simulink model "NewSpacecraft"  (R2020b)
settings: Solver=VariableStepAuto  StartTime=0.0  StopTime=10.0  RelTol=1e-3
undefined symbols (not defined in the file or in its folder): sim_constants
libraries: vrlib x2
settings Model: Creator=newpo  LastModifiedBy=newpo

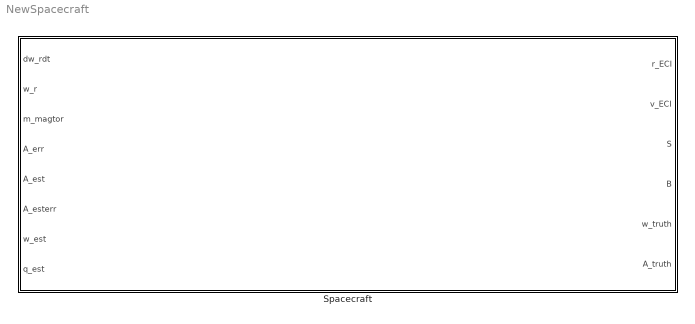
== system NewSpacecraft ==
  Spacecraft : Subsystem

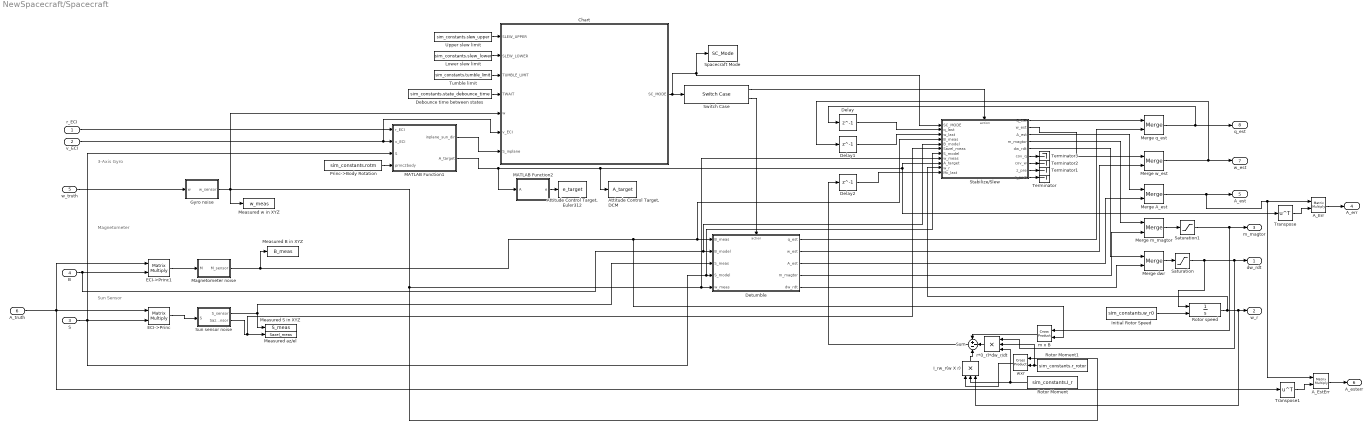
== system NewSpacecraft/Spacecraft ==
  note: Sun Sensor
  note: Magnetometer
  note: 3-Axis Gyro
  r_ECI : Inport
  v_ECI : Inport  Port=2
  S : Inport  Port=3
  B : Inport  Port=4
  w_truth : Inport  Port=5
  A_truth : Inport  Port=6
  A_Err : Product  Multiplication=Matrix(*)
  A_EstErr : Product  Multiplication=Matrix(*)
  "Attitude Control Target, DCM" : ToWorkspace  VariableName=A_target  SaveFormat=Timeseries  SampleTime=-1
  "Attitude Control Target, Euler312" : ToWorkspace  VariableName=e_target  SaveFormat=Timeseries  SampleTime=-1
  Chart : Stateflow chart  TreatAsAtomicUnit=on
  Debounce time between states : Constant  Value=sim_constants.state_debounce_time
  Delay : Delay  DelayLength=1  InitialCondition=sim_constants.q0
  Delay1 : Delay  DelayLength=1  InitialCondition=sim_constants.angvel0
  Delay2 : Delay  DelayLength=1  InitialCondition=[0;0;0]
  Detumble : Subsystem  TreatAsAtomicUnit=on
  ECI->Princ : Product  Multiplication=Matrix(*)
  ECI->Princ1 : Product  Multiplication=Matrix(*)
  Gyro noise : Subsystem
  I_rw_r(w X r) : Product  Inputs=3
  Initial Rotor Speed : Constant  Value=sim_constants.w_r0
  Lower slew limit : Constant  Value=sim_constants.slew_lower
  MATLAB Function1 : MATLAB Function  TreatAsAtomicUnit=on
  MATLAB Function2 : MATLAB Function  TreatAsAtomicUnit=on
  Magnetometer noise : Subsystem
  Measured B in XYZ : ToWorkspace  VariableName=B_meas  SaveFormat=Timeseries  SampleTime=-1
  Measured S in XYZ : ToWorkspace  VariableName=S_meas  SaveFormat=Timeseries  SampleTime=-1
  Measured az/el : ToWorkspace  VariableName=Sazel_meas  SaveFormat=Timeseries  SampleTime=-1
  Measured w in XYZ : ToWorkspace  VariableName=w_meas  SaveFormat=Timeseries  SampleTime=-1
  Merge A_est : Merge
  Merge dwr : Merge
  Merge m_magtor : Merge
  Merge q_est : Merge
  Merge w_est : Merge
  Princ->Body Rotation : Constant  Value=sim_constants.rotm
  Rotor Moment : Constant  Value=sim_constants.I_r
  Rotor Moment1 : Constant  Value=sim_constants.r_rotor
  Rotor speed : Integrator  InitialConditionSource=external  LimitOutput=on  UpperSaturationLimit=sim_constants.w_rmax  LowerSaturationLimit=-sim_constants.w_rmax
  Saturation : Saturate  UpperLimit=sim_constants.dw_rdtmax  LowerLimit=-sim_constants.dw_rdtmax
  Saturation1 : Saturate  UpperLimit=sim_constants.m_magtor_max  LowerLimit=-sim_constants.m_magtor_max
  Spacecraft Mode : ToWorkspace  VariableName=SC_Mode  SaveFormat=Timeseries  SampleTime=-1
  Stabilize/Slew : Subsystem  TreatAsAtomicUnit=on
  Sum : Sum  Inputs=+--
  Sun sensor noise : Subsystem
  Switch Case : SwitchCase  CaseConditions={[SCModeEnum.STABILIZE,SCModeEnum.SLEW],SCModeEnum.DETUMBLE}  ShowDefaultCase=off
  Terminator{,1..3} (4 alike) : Terminator
  Transpose : Math  Operator=transpose  SaturateOnIntegerOverflow=on
  Transpose1 : Math  Operator=transpose  SaturateOnIntegerOverflow=on
  Tumble limit : Constant  Value=sim_constants.tumble_limit
  Upper slew limit : Constant  Value=sim_constants.slew_upper
  m x B : vrlib/Utilities/Cross Product
  r*(I_r)*dw_r/dt : Product  Inputs=3
  wxr : vrlib/Utilities/Cross Product
  dw_rdt : Outport
  w_r : Outport  Port=2
  m_magtor : Outport  Port=3
  A_err : Outport  Port=4
  A_est : Outport  Port=5
  A_esterr : Outport  Port=6
  w_est : Outport  Port=7
  q_est : Outport  Port=8
  wires:
  Gyro noise/1(w_sensor) -> Chart/5(w), wxr/1, Stabilize/Slew/8(w_meas), Detumble/5(w_meas), Measured w in XYZ/1
  B/1 -> Stabilize/Slew/5(B_model), Detumble/2(B_model), ECI->Princ1/2
  Sun sensor noise/1(S_sensor) -> Measured S in XYZ/1, Detumble/3(S_meas)
  w_truth/1 -> Gyro noise/1(w)
  Sun sensor noise/2(Sazel_sensor) -> Stabilize/Slew/6(Sazel_meas), Measured az/el/1
  A_truth/1 -> Transpose1/1, ECI->Princ1/1, ECI->Princ/1
  ECI->Princ/1 -> Sun sensor noise/1(S)
  ECI->Princ1/1 -> Magnetometer noise/1(M)
  Princ->Body Rotation/1 -> MATLAB Function1/4(princ2body)
  MATLAB Function1/1(inplane_sun_dir) -> Chart/7(S_inplane)
  v_ECI/1 -> Chart/6(v_ECI), MATLAB Function1/2(v_ECI)
  r_ECI/1 -> MATLAB Function1/1(r_ECI)
  Chart/1(SC_MODE) -> Spacecraft Mode/1, Stabilize/Slew/1(SC_MODE), Switch Case/1
  Switch Case/2 -> Detumble/Action
  Magnetometer noise/1(M_sensor) -> m x B/2, Stabilize/Slew/4(B_meas), Detumble/1(B_meas), Measured B in XYZ/1
  S/1 -> Stabilize/Slew/7(S_model), Detumble/4(S_model), MATLAB Function1/3(S), ECI->Princ/2
  Switch Case/1 -> Stabilize/Slew/Action
  Merge q_est/1 -> Delay/1, q_est/1
  Delay/1 -> Stabilize/Slew/2(q_last)
  Detumble/1(q_est) -> Merge q_est/2
  Stabilize/Slew/1(q_est) -> Merge q_est/1
  Merge w_est/1 -> Delay1/1, w_est/1
  Delay1/1 -> Stabilize/Slew/3(w_last)
  Detumble/2(w_est) -> Merge w_est/2
  Stabilize/Slew/2(w_est) -> Merge w_est/1
  Rotor speed/1 -> I_rw_r(w X r)/3, w_r/1, Stabilize/Slew/10(w_r)
  Initial Rotor Speed/1 -> Rotor speed/2
  Merge dwr/1 -> Saturation/1
  Merge A_est/1 -> A_EstErr/1, A_Err/1, A_est/1
  Stabilize/Slew/3(A_est) -> Merge A_est/1
  Stabilize/Slew/4(m_magtor) -> Merge m_magtor/1
  Stabilize/Slew/5(dw_rdt) -> Merge dwr/1
  Detumble/3(A_est) -> Merge A_est/2
  Detumble/4(m_magtor) -> Merge m_magtor/2
  Detumble/5(dw_rdt) -> Merge dwr/2
  MATLAB Function1/2(A_target) -> MATLAB Function2/1(A), "Attitude Control Target, DCM"/1, Transpose/1, Stabilize/Slew/9(A_target)
  Stabilize/Slew/9(z_post) -> Terminator/1
  Stabilize/Slew/8(z_pre) -> Terminator1/1
  Stabilize/Slew/7(cov_w) -> Terminator2/1
  Stabilize/Slew/6(cov_q) -> Terminator3/1
  Transpose/1 -> A_Err/2
  A_Err/1 -> A_err/1
  Transpose1/1 -> A_EstErr/2
  A_EstErr/1 -> A_esterr/1
  Upper slew limit/1 -> Chart/1(SLEW_UPPER)
  Lower slew limit/1 -> Chart/2(SLEW_LOWER)
  Tumble limit/1 -> Chart/3(TUMBLE_LIMIT)
  Debounce time between states/1 -> Chart/4(TWAIT)
  MATLAB Function2/1(e) -> "Attitude Control Target, Euler312"/1
  Saturation/1 -> Rotor speed/1, r*(I_r)*dw_r/dt/1, dw_rdt/1
  Merge m_magtor/1 -> Saturation1/1
  Saturation1/1 -> m x B/1, m_magtor/1
  m x B/1 -> Sum/1
  Rotor Moment1/1 -> r*(I_r)*dw_r/dt/2, wxr/2
  Rotor Moment/1 -> I_rw_r(w X r)/2, r*(I_r)*dw_r/dt/3
  I_rw_r(w X r)/1 -> Sum/3
  wxr/1 -> I_rw_r(w X r)/1
  r*(I_r)*dw_r/dt/1 -> Sum/2
  Sum/1 -> Delay2/1
  Delay2/1 -> Stabilize/Slew/11(Mc_last)

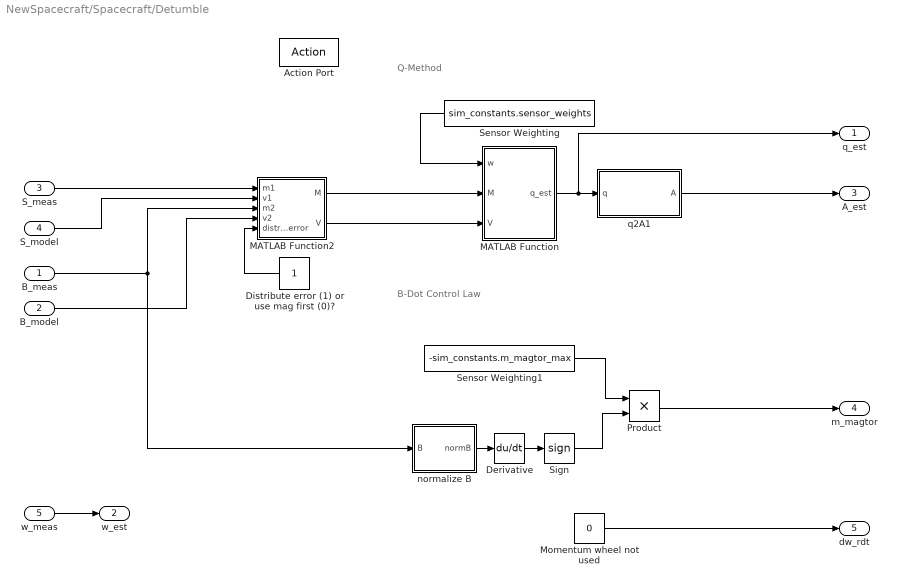
== system NewSpacecraft/Spacecraft/Detumble ==
  note: B-Dot Control Law
  note: Q-Method
  B_meas : Inport
  B_model : Inport  Port=2
  S_meas : Inport  Port=3
  S_model : Inport  Port=4
  w_meas : Inport  Port=5
  Action Port : ActionPort
  Derivative : Derivative  CoefficientInTFapproximation=0.1*2*pi*sim_constants.time_step
  Distribute error (1) or use mag first (0)? : Constant
  MATLAB Function : MATLAB Function  TreatAsAtomicUnit=on
  MATLAB Function2 : MATLAB Function  TreatAsAtomicUnit=on
  Momentum wheel not used : Constant  Value=0
  Product : Product
  Sensor Weighting : Constant  Value=sim_constants.sensor_weights
  Sensor Weighting1 : Constant  Value=-sim_constants.m_magtor_max
  Sign : Signum
  normalize B : MATLAB Function  TreatAsAtomicUnit=on
  q2A1 : MATLAB Function  TreatAsAtomicUnit=on
  q_est : Outport
  w_est : Outport  Port=2
  A_est : Outport  Port=3
  m_magtor : Outport  Port=4
  dw_rdt : Outport  Port=5
  wires:
  Sensor Weighting/1 -> MATLAB Function/1(w)
  S_meas/1 -> MATLAB Function2/1(m1)
  MATLAB Function2/2(V) -> MATLAB Function/3(V)
  q2A1/1(A) -> A_est/1
  MATLAB Function/1(q_est) -> q_est/1, q2A1/1(q)
  Distribute error (1) or use mag first (0)?/1 -> MATLAB Function2/5(distribute_error)
  B_meas/1 -> MATLAB Function2/3(m2), normalize B/1(B)
  MATLAB Function2/1(M) -> MATLAB Function/2(M)
  S_model/1 -> MATLAB Function2/2(v1)
  B_model/1 -> MATLAB Function2/4(v2)
  Derivative/1 -> Sign/1
  Sensor Weighting1/1 -> Product/1
  Sign/1 -> Product/2
  Product/1 -> m_magtor/1
  Momentum wheel not used/1 -> dw_rdt/1
  w_meas/1 -> w_est/1
  normalize B/1(normB) -> Derivative/1

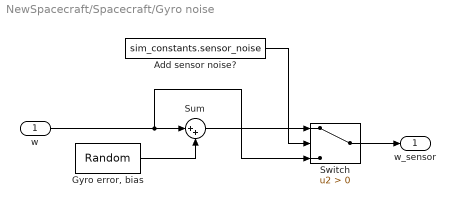
== system NewSpacecraft/Spacecraft/Gyro noise ==
  w : Inport
  Add sensor noise? : Constant  Value=sim_constants.sensor_noise
  "Gyro error, bias" : RandomNumber  Mean=sim_constants.gyro_bias  Variance=sim_constants.gyro_error  Seed=[0, 1, 2]  SampleTime=sim_constants.time_step
  Sum : Sum  Inputs=|++
  Switch : Switch  Criteria=u2 > Threshold
  w_sensor : Outport
  wires:
  "Gyro error, bias"/1 -> Sum/2
  w/1 -> Sum/1, Switch/3
  Switch/1 -> w_sensor/1
  Add sensor noise?/1 -> Switch/2
  Sum/1 -> Switch/1

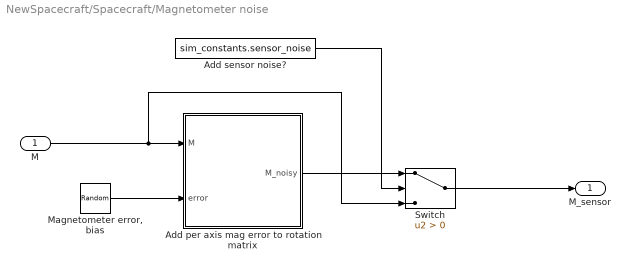
== system NewSpacecraft/Spacecraft/Magnetometer noise ==
  M : Inport
  Add per axis mag error to rotation matrix : MATLAB Function  TreatAsAtomicUnit=on
  Add sensor noise? : Constant  Value=sim_constants.sensor_noise
  "Magnetometer error, bias" : RandomNumber  Mean=sim_constants.mag_bias  Variance=sim_constants.mag_error  Seed=[6, 7, 8]  SampleTime=sim_constants.time_step
  Switch : Switch  Criteria=u2 > Threshold
  M_sensor : Outport
  wires:
  Add per axis mag error to rotation matrix/1(M_noisy) -> Switch/1
  Add sensor noise?/1 -> Switch/2
  M/1 -> Switch/3, Add per axis mag error to rotation matrix/1(M)
  "Magnetometer error, bias"/1 -> Add per axis mag error to rotation matrix/2(error)
  Switch/1 -> M_sensor/1

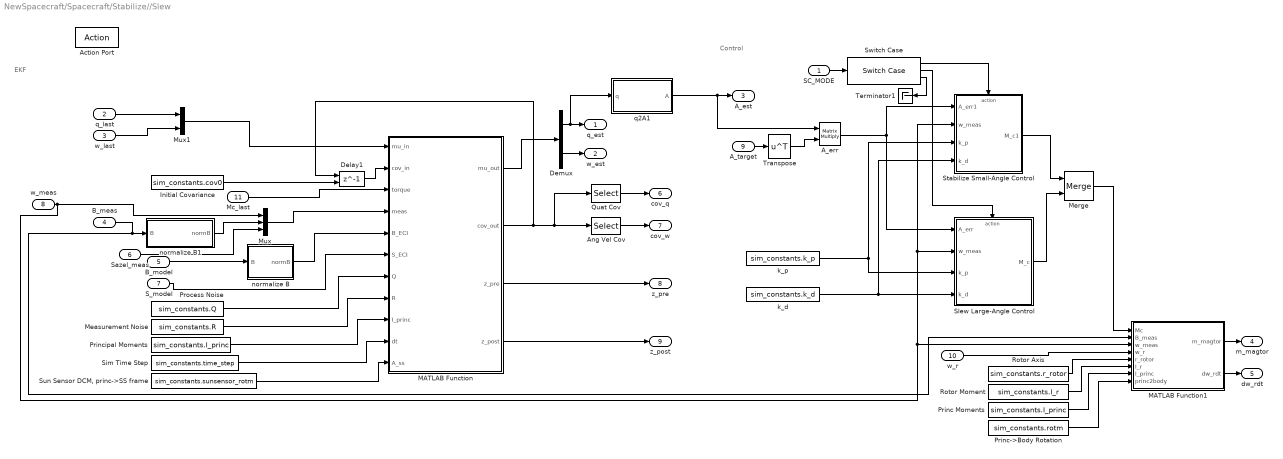
== system NewSpacecraft/Spacecraft/Stabilize//Slew ==
  note: Control
  note: EKF
  SC_MODE : Inport
  q_last : Inport  Port=2
  w_last : Inport  Port=3
  B_meas : Inport  Port=4
  B_model : Inport  Port=5
  Sazel_meas : Inport  Port=6
  S_model : Inport  Port=7
  w_meas : Inport  Port=8
  A_target : Inport  Port=9
  w_r : Inport  Port=10
  Mc_last : Inport  Port=11
  Action Port : ActionPort  InitializeStates=reset
  A_err : Product  Multiplication=Matrix(*)
  Ang Vel Cov : Selector  NumberOfDimensions=2  InputPortWidth=3  IndexOptions=Index vector (dialog),Index vector (dialog)  Indices=5:7,5:7  OutputSizes=1,1
  Delay1 : Delay  DelayLength=1  InitialConditionSource=Input port  InitialCondition=0
      settings: InputPortMap=u0,p4
  Demux : Demux  Outputs=[4, 3]
  Initial Covariance : Constant  Value=sim_constants.cov0
  MATLAB Function : MATLAB Function  TreatAsAtomicUnit=on
  MATLAB Function1 : MATLAB Function  TreatAsAtomicUnit=on
  Measurement Noise : Constant  Value=sim_constants.R
  Merge : Merge
  Mux : Mux  Inputs=3
  Mux1 : Mux  Inputs=2
  Princ Moments : Constant  Value=sim_constants.I_princ
  Princ->Body Rotation : Constant  Value=sim_constants.rotm
  Principal Moments : Constant  Value=sim_constants.I_princ
  Process Noise : Constant  Value=sim_constants.Q
  Quat Cov : Selector  NumberOfDimensions=2  InputPortWidth=3  IndexOptions=Index vector (dialog),Index vector (dialog)  Indices=1:4,1:4  OutputSizes=1,1
  Rotor Axis : Constant  Value=sim_constants.r_rotor
  Rotor Moment : Constant  Value=sim_constants.I_r
  Sim Time Step : Constant  Value=sim_constants.time_step
  Slew Large-Angle Control : Subsystem  TreatAsAtomicUnit=on
  Stabilize Small-Angle Control : Subsystem  TreatAsAtomicUnit=on
  "Sun Sensor DCM, princ->SS frame" : Constant  Value=sim_constants.sunsensor_rotm
  Switch Case : SwitchCase  CaseConditions={SCModeEnum.STABILIZE, SCModeEnum.SLEW}
  Terminator1 : Terminator
  Transpose : Math  Operator=transpose  SaturateOnIntegerOverflow=on
  k_d : Constant  Value=sim_constants.k_d
  k_p : Constant  Value=sim_constants.k_p
  normalize B : MATLAB Function  TreatAsAtomicUnit=on
  normalize B1 : MATLAB Function  TreatAsAtomicUnit=on
  q2A1 : MATLAB Function  TreatAsAtomicUnit=on
  q_est : Outport
  w_est : Outport  Port=2
  A_est : Outport  Port=3
  m_magtor : Outport  Port=4
  dw_rdt : Outport  Port=5
  cov_q : Outport  Port=6
  cov_w : Outport  Port=7
  z_pre : Outport  Port=8
  z_post : Outport  Port=9
  wires:
  "Sun Sensor DCM, princ->SS frame"/1 -> MATLAB Function/11(A_ss)
  Demux/2 -> w_est/1
  Sim Time Step/1 -> MATLAB Function/10(dt)
  Initial Covariance/1 -> Delay1/2
  MATLAB Function/4(z_post) -> z_post/1
  Sazel_meas/1 -> Mux/3
  Measurement Noise/1 -> MATLAB Function/8(R)
  MATLAB Function/3(z_pre) -> z_pre/1
  Ang Vel Cov/1 -> cov_w/1
  Principal Moments/1 -> MATLAB Function/9(I_princ)
  Process Noise/1 -> MATLAB Function/7(Q)
  MATLAB Function/1(mu_out) -> Demux/1
  Demux/1 -> q2A1/1(q), q_est/1
  w_meas/1 -> Mux/1, Stabilize Small-Angle Control/2(w_meas), Slew Large-Angle Control/2(w_meas), MATLAB Function1/3(w_meas)
  S_model/1 -> MATLAB Function/6(S_ECI)
  Mux/1 -> MATLAB Function/4(meas)
  Delay1/1 -> MATLAB Function/2(cov_in)
  B_meas/1 -> MATLAB Function1/2(B_meas), normalize B1/1(B)
  Quat Cov/1 -> cov_q/1
  MATLAB Function/2(cov_out) -> Delay1/1, Quat Cov/1, Ang Vel Cov/1
  B_model/1 -> normalize B/1(B)
  q_last/1 -> Mux1/1
  w_last/1 -> Mux1/2
  Mux1/1 -> MATLAB Function/1(mu_in)
  Mc_last/1 -> MATLAB Function/3(torque)
  Merge/1 -> MATLAB Function1/1(Mc)
  q2A1/1(A) -> A_err/1, A_est/1
  A_target/1 -> Transpose/1
  Transpose/1 -> A_err/2
  SC_MODE/1 -> Switch Case/1
  Switch Case/1 -> Stabilize Small-Angle Control/Action
  Stabilize Small-Angle Control/1(M_c1) -> Merge/1
  Slew Large-Angle Control/1(M_c) -> Merge/2
  MATLAB Function1/1(m_magtor) -> m_magtor/1
  MATLAB Function1/2(dw_rdt) -> dw_rdt/1
  Switch Case/2 -> Slew Large-Angle Control/Action
  A_err/1 -> Slew Large-Angle Control/1(A_err), Stabilize Small-Angle Control/1(A_err1)
  k_p/1 -> Slew Large-Angle Control/3(k_p), Stabilize Small-Angle Control/3(k_p)
  k_d/1 -> Stabilize Small-Angle Control/4(k_d), Slew Large-Angle Control/4(k_d)
  Switch Case/3 -> Terminator1/1
  normalize B/1(normB) -> MATLAB Function/5(B_ECI)
  normalize B1/1(normB) -> Mux/2
  w_r/1 -> MATLAB Function1/4(w_r)
  Rotor Axis/1 -> MATLAB Function1/5(r_rotor)
  Rotor Moment/1 -> MATLAB Function1/6(I_r)
  Princ->Body Rotation/1 -> MATLAB Function1/8(princ2body)
  Princ Moments/1 -> MATLAB Function1/7(I_princ)

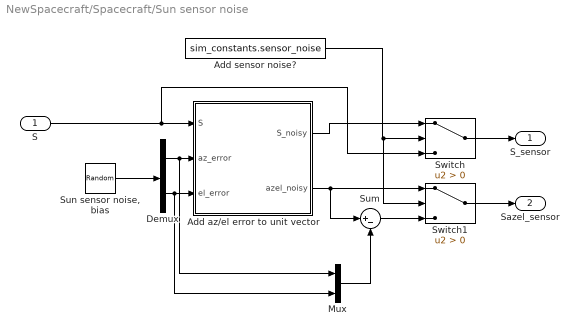
== system NewSpacecraft/Spacecraft/Sun sensor noise ==
  S : Inport
  Add az/el error to unit vector : MATLAB Function  TreatAsAtomicUnit=on
  Add sensor noise? : Constant  Value=sim_constants.sensor_noise
  Demux : Demux  Outputs=2
  Mux : Mux  Inputs=2
  Sum : Sum  Inputs=|+-
  "Sun sensor noise, bias" : RandomNumber  Mean=sim_constants.ss_bias  Variance=sim_constants.ss_error  Seed=[4, 5]  SampleTime=sim_constants.time_step
  Switch : Switch  Criteria=u2 > Threshold
  Switch1 : Switch  Criteria=u2 > Threshold
  S_sensor : Outport
  Sazel_sensor : Outport  Port=2
  wires:
  Demux/1 -> Mux/1, Add az/el error to unit vector/2(az_error)
  Demux/2 -> Mux/2, Add az/el error to unit vector/3(el_error)
  "Sun sensor noise, bias"/1 -> Demux/1
  S/1 -> Switch/3, Add az/el error to unit vector/1(S)
  Switch/1 -> S_sensor/1
  Add az/el error to unit vector/1(S_noisy) -> Switch/1
  Add sensor noise?/1 -> Switch1/2, Switch/2
  Add az/el error to unit vector/2(azel_noisy) -> Sum/1, Switch1/1
  Mux/1 -> Sum/2
  Sum/1 -> Switch1/3
  Switch1/1 -> Sazel_sensor/1

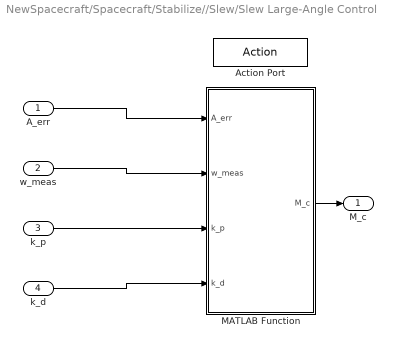
== system NewSpacecraft/Spacecraft/Stabilize//Slew/Slew Large-Angle Control ==
  A_err : Inport
  w_meas : Inport  Port=2
  k_p : Inport  Port=3
  k_d : Inport  Port=4
  Action Port : ActionPort
  MATLAB Function : MATLAB Function  TreatAsAtomicUnit=on
  M_c : Outport
  wires:
  A_err/1 -> MATLAB Function/1(A_err)
  w_meas/1 -> MATLAB Function/2(w_meas)
  k_p/1 -> MATLAB Function/3(k_p)
  k_d/1 -> MATLAB Function/4(k_d)
  MATLAB Function/1(M_c) -> M_c/1

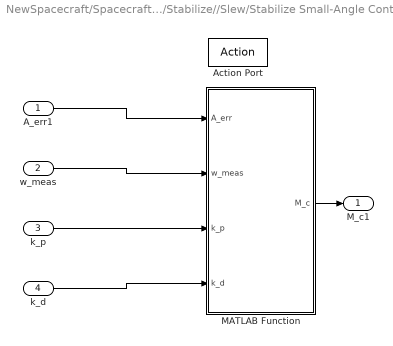
== system NewSpacecraft/Spacecraft/Stabilize//Slew/Stabilize Small-Angle Control ==
  A_err1 : Inport
  w_meas : Inport  Port=2
  k_p : Inport  Port=3
  k_d : Inport  Port=4
  Action Port : ActionPort
  MATLAB Function : MATLAB Function  TreatAsAtomicUnit=on
  M_c1 : Outport
  wires:
  MATLAB Function/1(M_c) -> M_c1/1
  A_err1/1 -> MATLAB Function/1(A_err)
  w_meas/1 -> MATLAB Function/2(w_meas)
  k_d/1 -> MATLAB Function/4(k_d)
  k_p/1 -> MATLAB Function/3(k_p)

== matlab function NewSpacecraft/Spacecraft/MATLAB Function1 ==
  data: inplane_sun_dir output; r_ECI input; A_target output; v_ECI input; S input; princ2body input
function [inplane_sun_dir, A_target] = target_attitude(r_ECI, v_ECI, S, princ2body)
    % Calculate in-plane sun direction
    h = cross(r_ECI, v_ECI); % angular momentum vector, normal to orbital plane
    h = h/norm(h); % unitize
    inplane_sun_dir = S - dot(h,S)*h; % get in-plane sun direction
    if all(abs(inplane_sun_dir) < 1E-6)% if sun direction is perpendicular to orbital plane 
        inplane_sun_dir = r_ECI/norm(r_ECI); % just assume sun is in radial direction
    else
        inplane_sun_dir = inplane_sun_dir/norm(inplane_sun_dir);
    end
    A_body2ECI = zeros(3);
    if dot(v_ECI, S) < 0 % if moving away from the sun
        A_body2ECI(:,1) = h; % align body x axis with orbit plane normal
        A_body2ECI(:,3) = -inplane_sun_dir; % align body z to be along projection of -S in orbit plane (SRP thrusting in-plane)
        A_body2ECI(:,2) = cross( A_body2ECI(:,2) ,  A_body2ECI(:,3) ); % y completes triad
    else
        A_body2ECI(:,1) = h; % align body x axis with orbit plane normal
        A_body2ECI(:,2) = inplane_sun_dir; % align body y to be along projection of S in orbit plane (no thrusting)
        A_body2ECI(:,3) = cross( A_body2ECI(:,1) ,  A_body2ECI(:,2) ); % z completes triad
    end
    A_target = A_body2ECI*(princ2body.'); % princ->body->ECI
    A_target = A_target.'; % ECI->Princ(target)
end

== matlab function NewSpacecraft/Spacecraft/Detumble/MATLAB Function2 ==
  data: m1 input; v1 input; M output; m2 input; v2 input; V output; distribute_error input
function [M, V] = makeMV(m1, v1, m2, v2, distribute_error)

    if distribute_error
        m1_av = (m1 + m2)/2;
        m2_av = (m1 - m2)/2;
        m1 = m1_av; m2 = m2_av;
        
        v1_av = (v1 + v2)/2;
        v2_av = (v1 - v2)/2;
        v1 = v1_av; v2 = v2_av;
    end
        
    q = cross(m1,m2);
    q = q/norm(q);
    r = cross(m1,q);
    M = [m1, q, r];

    qv = cross(v1,v2);
    qv = qv/norm(qv);
    rv = cross(v1,qv);
    V = [v1, qv, rv];

end

== matlab function NewSpacecraft/Spacecraft/Stabilize//Slew/MATLAB Function ==
  data: mu_in input; mu_out output; cov_in input; torque input; meas input; B_ECI input; S_ECI input; Q input; R input; I_princ input; dt input; cov_out output; z_pre output; z_post output; A_ss input
%% satEKF
% Extended Kalman filter for satellite attitude state estimation.
% mu_in : the current estimated state mean, in the form
%           (q, w, bw, bB, bS)^T
%           where q is the quaternion, w is the principal axes angular
%           velocity, bw is the gyroscopic sensor bias, bB is the magnetic
%           sensor bias, and bS is the azimuth/elevation sun sensor bias.
% cov_in : the current covariance matrix
% torque : the input torque to the system at the current time step
% meas : the measurement of the current state
% B_ECI : the modeled magnetic field vector in inertial coordinates at current time
% S_ECI: the modeled sun-pointing vector in intertial coordinates at current time 
% Q : the process noise matrix
% R : the measurement noise matrix
% I_princ : the principal moments of inertia corresponding to principal XYZ
% dt : the time step
% A_ss : the rotation from principal axes to sun sensor frame
function [mu_out, cov_out, z_pre, z_post] = satEKF_nobias(mu_in, cov_in, torque, meas, B_ECI, S_ECI, Q, R, I_princ, dt, A_ss)
    q = mu_in(1:4); % quaternion
    q = q/norm(q);
    w = mu_in(5:7); % angular velocity in princ
    
    At = A(q,w,I_princ,dt);
    %% Predict - use non-linear function to predict mean, linearized info for cov
    mu_p = f(mu_in,torque,I_princ,dt); % get predicted state from non-linear eq
    cov_p = At*cov_in*(At.') + Q;
    A_p = q2A(mu_p(1:4)/norm(mu_p(1:4))); % get rotation matrix of predicted state
    meas_p = g(mu_p,A_p*B_ECI,A_p*S_ECI,A_ss); % predicted measurement
    z_pre = z(meas, meas_p); % pre-fit residual (diff between real and predicted)
    %% Update - use predicted states to compute Kalman gain and final update
    % Update state using sensitivity matrix
    q_p = mu_p(1:4)/norm(mu_p(1:4));
    Ct = C(q_p,q2A(q_p),B_ECI,S_ECI,A_ss); % Sensitivity matrix
    K = cov_p*(Ct.')/(Ct*cov_p*(Ct.') + R) ; % Kalman Gain
    mu_out = mu_p + K*z_pre;
    T = (eye(7) - K*Ct);
    cov_out = T*cov_p*(T.') + K*R*(K.');
    A_f = q2A(mu_out(1:4)/norm(mu_out(1:4)));
    z_post = z(meas, g(mu_out,A_f*B_ECI,A_f*S_ECI,A_ss));  % post-fit residual (diff between real and estimated)
end
% Helper Functions
    function O = Omega(w)
        % Returns Omega(w), the rate relation such that dw/dt = 0.5*Omega*q
        O = [0 w(3) -w(2) w(1);
             -w(3) 0 w(1) w(2);
             w(2) -w(1) 0 w(3);
             -w(1) -w(2) -w(3) 0];
    end
    function L = Lambda(q)
        % Returns Lambda(q), the rate relation such that dw/dt = 0.5*Lambda*w
        L = [q(4) -q(3) q(2);
             q(3) q(4) -q(1);
             -q(2) q(1) q(4);
             -q(1) -q(2) -q(3) ];
    end
    function D = Delta(w,I)
        % Returns Delta(w), the partial derivative of the Euler equations
        % wrt angular velocity.
        D = [0 (I(2)-I(3))/I(1)*w(3) (I(2)-I(3))/I(1)*w(2);
             (I(3)-I(1))/I(2)*w(3) 0 (I(3)-I(1))/I(2)*w(1);
             (I(1)-I(2))/I(3)*w(2) (I(1)-I(2))/I(3)*w(1) 0 ];
    end
    function G = Gamma(q,V)
        % Returns Gamma(q,V), the partial derivative of A(q)*V wrt to the
        % quaternion, for some vector V in ECI.
        q = q/norm(q);
        qvec = q(1:3);
        a = [-q(2);q(1);-q(4)];
        b = [-q(3);q(4);q(1)];
        c = [q(4); q(3); -q(2)];
        G = 2*[dot(qvec,V) dot(a,V) dot(b,V) dot(c,V);
               dot(-a,V) dot(qvec,V) dot(-c,V) dot(b,V);
               dot(-b,V) dot(c,V) dot(qvec,V) dot(-a,V) ];
    end
    function Mt = M(S)
        Mt = [atan2(S(2),S(1)); acos(S(3))];
    end
    function Mt = Mtilde(S)
        S12 = S(1)^2 + S(2)^2;
        Mt = [-S(2)/S12 S(1)/S12 0; 0 0 -1/sqrt(1-S(3)^2)];
    end
    function xout = f(x,torque,I,dt)
        % Dynamics function such that x_{t+1} = f(x_t, u_t)
        q = x(1:4);
        w = x(5:7);
        s = eye(7); 
        normq = norm(q);
        s(1:4,1:4) = eye(4)/normq;
        xout = s*(x + dt*[0.5*Omega(w)*q ; (torque - cross(w,I.*w))./I]);
    end
    function At = A(q,w,I,dt)
        % Jacobian of dynamics
        normq = norm(q);
        q = q/normq;
        s = eye(7); 
        b = diag((normq^2)*ones(4,1)-(q.^2)); % b = d/dq of (q/norm(q))
        b(1,2:4) = -q(2:4).' * q(1) ;
        b(2,[1 3 4]) = -q([1 3 4]).' * q(2) ;
        b(3,[1 2 4]) = -q([1 2 4]).' * q(3) ;
        b(2,[1 2 3]) = -q([1 2 3]).' * q(4) ;
        b = b/(normq^3);
        s(1:4,1:4) = b;
        At = s + dt*[0.5*Omega(w).*b 0.5*Lambda(q)/normq;
              zeros(3,4) Delta(w,I) ];
    end
    function y = g(x,B_XYZ,S_XYZ,A_ss)
        % Measurement function such that y_t = g(x_t,u_t)
        % A is the computed rotation matrix taken from the first four
        % elements of x
        y = zeros(8,1);
        y(1:3) = x(5:7); % angular velocity measurement, w/ bias
        y(4:6) = B_XYZ ; % magnetic field strength in XYZ, w/ bias
        y(7:8) = M(A_ss*S_XYZ); % sun az/el in sensor frame w/ bias
        y(7) = mod(y(7),2*pi); % wrap azimuth to 2*pi
        % Limit to elevation to (-90, 90)
        if y(8) < -pi/2
            y(8) = -pi - y(8);
            y(7) = mod(y(7) + pi, 2*pi);
        elseif y(8) > pi/2 
            y(8) = pi - y(8);
            y(7) = mod(y(7) + pi, 2*pi);
        end
    end
    function Ct = C(q,Aq,B_ECI,S_ECI,A_ss)
        S_xyz = Aq*S_ECI;
        Ct = [zeros(3,4) eye(3);
              Gamma(q,B_ECI) zeros(3);
              Mtilde(A_ss*S_xyz)*A_ss*Gamma(q,S_ECI) zeros(2,3)];
    end
    function zt = z(y, g)
        zt = y-g;
        azy = y(7); ely = y(8);
        azg = g(7); elg = g(8);
        % check if azimuth is near the turn-over point 2*pi->0
        if azy < pi/2 && azg > 3*pi/2
           azg = azg - 2*pi;
        elseif azy > 3*pi/2 && azg < pi/2
           azy = azy - 2*pi;
        end
        % check that azimuths aren't near-opposite, if so, flip
        if abs(azy-azg) > pi/0
            azg = mod(azg+pi, 2*pi); % flip azg
            if elg > 0
               elg = pi - elg;
            else
               elg = -pi - elg;
            end
        end
        zt(7:8) = [azy-azg; ely-elg];
    end

== matlab function NewSpacecraft/Spacecraft/Stabilize//Slew/MATLAB Function1 ==
  data: Mc input; m_magtor output; B_meas input; w_meas input; w_r input; r_rotor input; I_r input; I_princ input; princ2body input; dw_rdt output
function [m_magtor, dw_rdt] = Mc2magdw(Mc, B_meas, w_meas, w_r, r_rotor, I_r, I_princ, princ2body)
    % Calculations done in body frame, then returned to spacecraft frame
    % Assumes we have two orthogonal
    % magnetorqers along the body Y and Z axes.
    Mc = Mc + cross(w_meas,I_princ.*w_meas); % add cross term
    Mc = Mc + I_r*w_r*cross(w_meas,r_rotor); % add momentum wheel term
    B = princ2body*B_meas;
    rbody = princ2body*r_rotor;
    control = [rbody, [B(3) -B(2); 0 B(1); -B(1) 0]];
    control = control\(princ2body*Mc); % calculate necessary input for desired torque
    control = (princ2body.')*control; % return to principal coords
    dw_rdt = -control(1)/I_r;
    m_magtor = zeros(3,1);
    m_magtor(2:3) = control(2:3);
end

== matlab function NewSpacecraft/Spacecraft/Stabilize//Slew/Slew Large-Angle Control/MATLAB Function ==
  data: A_err input; M_c output; w_meas input; k_p input; k_d input
function M_c = LargeAngleControl(A_err,w_meas,k_p,k_d)
    A = 0.5*[A_err(2,3)-A_err(3,2);A_err(3,1)-A_err(1,3);A_err(1,2)-A_err(2,1)];
    M_c = -k_p.*A - k_d.*w_meas;
end

== matlab function NewSpacecraft/Spacecraft/Stabilize//Slew/Stabilize Small-Angle Control/MATLAB Function ==
  data: A_err input; M_c output; w_meas input; k_p input; k_d input
function M_c = LargeAngleControl(A_err,w_meas,k_p,k_d)
    A = 0.5*[A_err(2,3)-A_err(3,2);A_err(3,1)-A_err(1,3);A_err(1,2)-A_err(2,1)];
    M_c = -k_p.*A - k_d.*w_meas;
end

== matlab function NewSpacecraft/Spacecraft/Stabilize//Slew/q2A1 ==
  data: q input; A output
%% q2A - Calculate cosine matrix from q (or euler angles)
function A = q2A(q)
    qvec = reshape(q(1:3),3,1);
    skewq = [0 -qvec(3) qvec(2); qvec(3) 0 -qvec(1) ; -qvec(2) qvec(1) 0];
    A = (q(4)^2 - sum(qvec.^2))*eye(3) + 2*qvec*(qvec') - 2*q(4)*skewq ;
end

== matlab function NewSpacecraft/Spacecraft/Detumble/MATLAB Function ==
  data: q_est output; w input; M input; V input
function q_est = qmethod(w,M,V)
    w = reshape(w,1,[]); % row vec
    W = M.*(ones(size(M,1),1)*sqrt(w)); % Wi = sqrt(wi)*Mi
    U = V.*(ones(size(V,1),1)*sqrt(w)); % Ui = sqrt(wi)*Vi
    B = W*(U.');
    S = B + B.' ;
    Z = [ B(2,3)-B(3,2) ; B(3,1)-B(1,3) ; B(1,2)-B(2,1) ];
    sig = trace(B);
    K = [ S-sig*eye(size(S)) ; Z.' ];
    K = [K, [Z; sig]];
    [eVec, e] = eig(K);
    e = diag(e); % take to vector
    [~, maxi] = max(e);
    q_est = real(eVec(:,maxi)); % have to protect against complex, simulink worries
    q_est = q_est/norm(q_est); % normalize
end

== matlab function NewSpacecraft/Spacecraft/Detumble/q2A1 ==
  data: q input; A output
%% q2A - Calculate cosine matrix from q (or euler angles)
function A = q2A(q)
    qvec = reshape(q(1:3),3,1);
    skewq = [0 -qvec(3) qvec(2); qvec(3) 0 -qvec(1) ; -qvec(2) qvec(1) 0];
    A = (q(4)^2 - sum(qvec.^2))*eye(3) + 2*qvec*(qvec') - 2*q(4)*skewq ;
end

== matlab function NewSpacecraft/Spacecraft/MATLAB Function2 ==
  data: A input; e output
function e = A2e(A)
    A( abs(A) > 1 ) = 1;
    A( abs(A) < -1 ) = -1;
    e = [ atan2(A(1,2),A(2,2)) ;
          -asin(A(3,2))         ;
          atan2(A(3,1),A(3,3)) ; ];
end

== matlab function NewSpacecraft/Spacecraft/Detumble/normalize B ==
  data: B input; normB output
function normB = normalize(B)
    normB = B./norm(B);
end

== matlab function NewSpacecraft/Spacecraft/Sun sensor noise/Add az//el error to unit vector ==
  data: S input; az_error input; el_error input; S_noisy output; azel_noisy output
function [S_noisy, azel_noisy] = SS_error(S, az_error, el_error)
    % Error in deg.
    S = S/norm(S); % ensure normalization
    az = atan2(S(2), S(1)) + az_error;
    el = acos(S(3)) + el_error;
    
    % Limit to [0, 360], (-90, 90)
    az = mod(az, 2*pi); % azimuth is 0 to 2*pi
    if el < -pi/2
        el = -pi - el;
        az = mod(az + pi, 2*pi);
    elseif el > pi/2 
        el = pi - el;
        az = mod(az + pi, 2*pi);
    end
    
    x = cos(az)*sin(el);
    y = sin(az)*sin(el);
    z = cos(el);
    
    S_noisy = [x; y; z];
    azel_noisy = [az; el];
end

== matlab function NewSpacecraft/Spacecraft/Magnetometer noise/Add per axis mag error to rotation matrix ==
  data: M input; error input; M_noisy output
function M_noisy = Mag_error(M, error)
    % Add error
    M_noisy = M + reshape(error,3,1);
end

== matlab function NewSpacecraft/Spacecraft/Stabilize//Slew/normalize B ==
  data: B input; normB output
function normB = normalize(B)
    normB = B./norm(B);
end

== matlab function NewSpacecraft/Spacecraft/Stabilize//Slew/normalize B1 ==
  data: B input; normB output
function normB = normalize(B)
    normB = B./norm(B);
end

== stateflow chart NewSpacecraft/Spacecraft/Chart ==
  state SC_state [parallel]
    settings: executionOrder=1
    state stabilize
      entry:SC_MODE=STABILIZE;
    state slew
      entry: SC_MODE=SLEW;
    state detumble
      entry: SC_MODE = DETUMBLE;
    stabilize -> SC_state.slew [order 1] : Slew
    SC_state.slew -> stabilize [order 1] : Stabilize
    detumble -> stabilize : Stabilize
    stabilize -> detumble [order 2] : Detumble
    SC_state.slew -> detumble [order 2] : Detumble
    (default) -> detumble
  state SC_selectstate [parallel]
    settings: executionOrder=2
    state steady_state
    state stop_detumble
    state slew
    state do_detumble
    state start_detumble
    steady_state -> SC_selectstate.slew [order 2] : [abs(dot(v_ECI/norm(v_ECI),S_inplane))<SLEW_LOWER]
        | {send(Slew,SC_state)}
    stop_detumble -> steady_state [order 2] : after(TWAIT,sec)
        | [norm(w)<TUMBLE_LIMIT]
        | {send(Stabilize,SC_state)}
    SC_selectstate.slew -> steady_state [order 1] : [abs(dot(v_ECI/norm(v_ECI),S_inplane))>SLEW_UPPER]
        | {send(Stabilize,SC_state)}
    start_detumble -> steady_state [order 2] : [norm(w) < TUMBLE_LIMIT]
    steady_state -> start_detumble [order 1] : [norm(w) > TUMBLE_LIMIT]
    stop_detumble -> do_detumble [order 1] : [norm(w) > TUMBLE_LIMIT]
    do_detumble -> stop_detumble : [norm(w) < TUMBLE_LIMIT]
    SC_selectstate.slew -> start_detumble [order 2] : [norm(w) > TUMBLE_LIMIT]
    (default) -> do_detumble
    start_detumble -> do_detumble [order 1] : after(TWAIT,sec)
        | [norm(w)>TUMBLE_LIMIT]
        | {send(Detumble,SC_state)}
  data: SLEW_UPPER input; SLEW_LOWER input; TUMBLE_LIMIT input; TWAIT input =1; w input; v_ECI input; S_inplane input; SC_MODE output Enum: SCModeEnum
  events: Stabilize local FUNCTION_CALL_EVENT; Slew local FUNCTION_CALL_EVENT; Detumble local FUNCTION_CALL_EVENT
